simulink model "Fixed_Channel_Model_4_Channels"  (R2023a)
settings: Solver=ode23tb  StartTime=0.0  StopTime=3  RelTol=1e-3
libraries: dspfdesign x5, dspsrcs4 x4, dspvision x2
settings Model: Creator=zacha  LastModifiedBy=zacha
settings DebuggingCC: UnconnectedInputMsg=warning  UnconnectedOutputMsg=warning  UnconnectedLineMsg=warning
settings ModelReferenceCC: EnableRefExpFcnMdlSchedulingChecks=on
settings RTWCC: DLArmComputeVersion=19.05

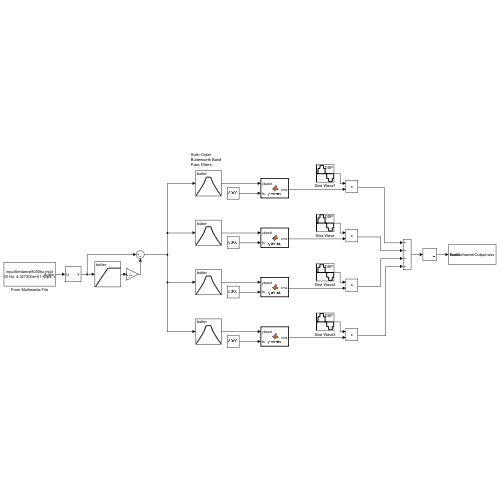
[thumbnail: Simulink's stored preview of the top-level diagram]
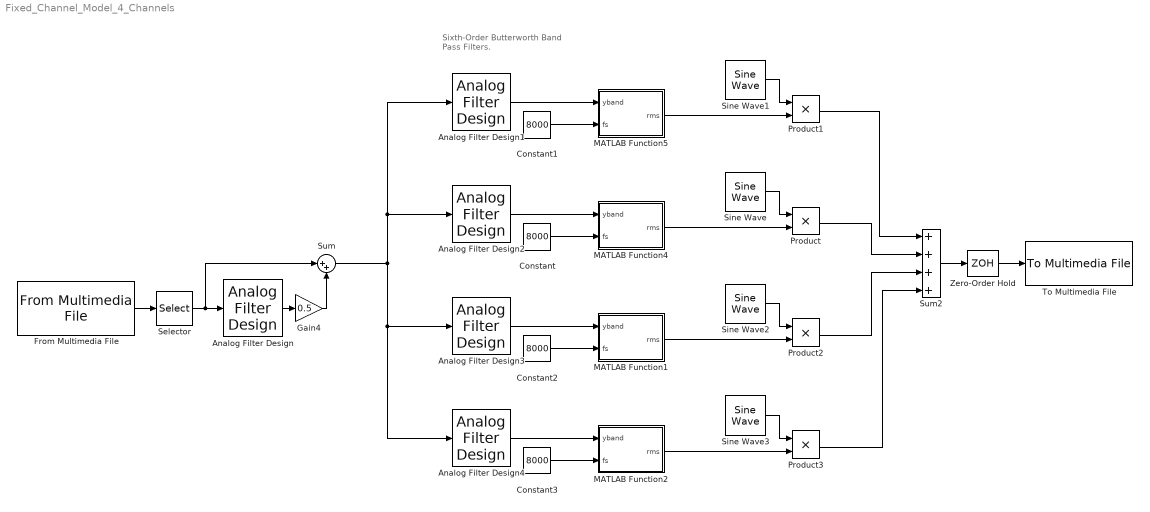
== system Fixed_Channel_Model_4_Channels ==
  note: Sixth-Order Butterworth Band Pass Filters.
  Analog Filter Design : dspfdesign/Analog Filter Design  method=Butterworth  filttype=Highpass  N=6  Wlo=7539.82236  Whi=80  Rp=2  Rs=40
  Analog Filter Design1 : dspfdesign/Analog Filter Design  method=Butterworth  filttype=Bandpass  N=6  Wlo=1570.796325  Whi=3476.7440370873  Rp=2  Rs=40
  Analog Filter Design2 : dspfdesign/Analog Filter Design  method=Butterworth  filttype=Bandpass  N=6  Wlo=3476.7440370873  Whi=7690.6188072  Rp=2  Rs=40
  Analog Filter Design3 : dspfdesign/Analog Filter Design  method=Butterworth  filttype=Bandpass  N=6  Wlo=7690.6188072  Whi=17032.45871124  Rp=2  Rs=40
  Analog Filter Design4 : dspfdesign/Analog Filter Design  method=Butterworth  filttype=Bandpass  N=6  Wlo=17032.45871124  Whi=37699.1118  Rp=2  Rs=40
  Constant{,1..3} (4 alike) : Constant  Value=8000
  From Multimedia File : dspvision/From Multimedia File  inputFilename=C:\Users\zacha\Desktop\Cochlear\Media\inputSentance8000hz.mp3  readRange=[1 Inf]  loop=on  numPlays=1  outputStreams=Audio only  videoDataType=single  audioDataType=double  inheritSampleTime=off  userDefinedSampleTime=1/8000  noAudioOutput=off  isIntensityVideo=off  fourcc=RGB  colorVideoFormat=Separate color signals  outputEOF=off  dataOrg=Column-major  audioFrameSize=1  computeAudioFrameSize=off  outSamplingMode=Sample based
      settings: LibrarySourceBlock=dspsrcs4/From Multimedia File
  Gain4 : Gain  Gain=0.5
  MATLAB Function1 : MATLAB Function  TreatAsAtomicUnit=on
  MATLAB Function2 : MATLAB Function  TreatAsAtomicUnit=on
  MATLAB Function4 : MATLAB Function  TreatAsAtomicUnit=on
  MATLAB Function5 : MATLAB Function  TreatAsAtomicUnit=on
  Product{,1..3} (4 alike) : Product
  Selector : Selector  NumberOfDimensions=2  InputPortWidth=3  IndexOptions=Select all,Index vector (dialog)  Indices=[2],1  OutputSizes=1,1
  Sine Wave : dspsrcs4/Sine Wave  Amplitude=1  Frequency=889.042915620874  Phase=0  SampleMode=Discrete  OutComplex=Real  CompMethod=Trigonometric fcn  TableSize=Speed  SampleTime=1/8000  SamplesPerFrame=1  ResetState=Restart at time zero  OutputFrames=off  dataType=double  wordLen=16  udDataType=sfix(16)  fracBitsMode=Best precision  numFracBits=15  OutDataTypeStr=double  LastOutDataTypeStr=double
  Sine Wave1 : dspsrcs4/Sine Wave  Amplitude=1  Frequency=401.670479925080  Phase=0  SampleMode=Discrete  OutComplex=Real  CompMethod=Trigonometric fcn  TableSize=Speed  SampleTime=1/8000  SamplesPerFrame=1  ResetState=Restart at time zero  OutputFrames=off  dataType=double  wordLen=16  udDataType=sfix(16)  fracBitsMode=Best precision  numFracBits=15  OutDataTypeStr=double  LastOutDataTypeStr=double
  Sine Wave2 : dspsrcs4/Sine Wave  Amplitude=1  Frequency=1967.77544111056  Phase=0  SampleMode=Discrete  OutComplex=Real  CompMethod=Trigonometric fcn  TableSize=Speed  SampleTime=1/8000  SamplesPerFrame=1  ResetState=Restart at time zero  OutputFrames=off  dataType=double  wordLen=16  udDataType=sfix(16)  fracBitsMode=Best precision  numFracBits=15  OutDataTypeStr=double  LastOutDataTypeStr=double
  Sine Wave3 : dspsrcs4/Sine Wave  Amplitude=1  Frequency=4355.40300541476  Phase=0  SampleMode=Discrete  OutComplex=Real  CompMethod=Trigonometric fcn  TableSize=Speed  SampleTime=1/8000  SamplesPerFrame=1  ResetState=Restart at time zero  OutputFrames=off  dataType=double  wordLen=16  udDataType=sfix(16)  fracBitsMode=Best precision  numFracBits=15  OutDataTypeStr=double  LastOutDataTypeStr=double
  Sum : Sum  Inputs=|++
  Sum2 : Sum  Inputs=++++
  To Multimedia File : dspvision/To Multimedia File  outputFilename=C:\Users\zacha\Desktop\Cochlear\Media\fixed4channelOutput.wav  streamSelection=Audio only  videoCompressor=None (uncompressed)  audioCompressor=None (uncompressed)  imagePorts=Separate color signals  fileType=WAV  audioDatatype=16-bit integer  fourcc=RGB  videoQuality=75  mj2000CompFactor=10
      settings: LibrarySourceBlock=dspsnks4/To Multimedia File
  Zero-Order Hold : ZeroOrderHold  SampleTime=-1
  wires:
  Analog Filter Design2/1 -> MATLAB Function4/1(yband)
  Constant/1 -> MATLAB Function4/2(fs)
  MATLAB Function4/1(rms) -> Product/2
  Sine Wave/1 -> Product/1
  Product/1 -> Sum2/2
  Product1/1 -> Sum2/1
  Sine Wave1/1 -> Product1/1
  Analog Filter Design1/1 -> MATLAB Function5/1(yband)
  MATLAB Function5/1(rms) -> Product1/2
  Constant1/1 -> MATLAB Function5/2(fs)
  Selector/1 -> Analog Filter Design/1, Sum/1
  Sine Wave2/1 -> Product2/1
  Analog Filter Design3/1 -> MATLAB Function1/1(yband)
  MATLAB Function1/1(rms) -> Product2/2
  Constant2/1 -> MATLAB Function1/2(fs)
  Sum/1 -> Analog Filter Design1/1, Analog Filter Design2/1, Analog Filter Design4/1, Analog Filter Design3/1
  Sine Wave3/1 -> Product3/1
  MATLAB Function2/1(rms) -> Product3/2
  Analog Filter Design4/1 -> MATLAB Function2/1(yband)
  Constant3/1 -> MATLAB Function2/2(fs)
  Product2/1 -> Sum2/3
  Product3/1 -> Sum2/4
  Sum2/1 -> Zero-Order Hold/1
  Zero-Order Hold/1 -> To Multimedia File/1
  From Multimedia File/1 -> Selector/1
  Analog Filter Design/1 -> Gain4/1
  Gain4/1 -> Sum/2

== matlab function Fixed_Channel_Model_4_Channels/MATLAB Function2 ==
  data: yband input; rms output; fs input
function rms = getrms(yband,fs)

    y = abs(yband); %rectifying it makes it sound bad

    [b,a] = butter(2,400/(fs/2));

    z = filter(b,a,y); %this filter also makes it sound bad

    windowsize = round(4/(1000/fs)); %rms computed every 4ms = windowsize samples

    [yupper,ylower] = envelope(yband,windowsize,'rms'); %changed to yband here

    %envelope(z,windowsize,'rms');

    rms = yupper;
end

== matlab function Fixed_Channel_Model_4_Channels/MATLAB Function4 ==
  data: yband input; rms output; fs input
function rms = getrms(yband,fs)

    y = abs(yband); %rectifying it makes it sound bad

    [b,a] = butter(2,400/(fs/2));

    z = filter(b,a,y); %this filter also makes it sound bad

    windowsize = round(4/(1000/fs)); %rms computed every 4ms = windowsize samples

    [yupper,ylower] = envelope(yband,windowsize,'rms'); %changed to yband here

    %envelope(z,windowsize,'rms');

    rms = yupper;
end

== matlab function Fixed_Channel_Model_4_Channels/MATLAB Function5 ==
  data: yband input; rms output; fs input
function rms = getrms(yband,fs)

    %y = abs(yband); %rectifying it makes it sound bad

    [b,a] = butter(2,400/(fs/2));

    %z = filter(b,a,y); %this filter also makes it sound bad

    windowsize = round(4/(1000/fs)); %rms computed every 4ms = windowsize samples

    [yupper,ylower] = envelope(yband,windowsize,'rms'); %changed to yband here

    %[yupper,ylower] = envelope(z,windowsize,'rms');

    rms = yupper;
end

== matlab function Fixed_Channel_Model_4_Channels/MATLAB Function1 ==
  data: yband input; rms output; fs input
function rms = getrms(yband,fs)

    y = abs(yband); %rectifying it makes it sound bad

    [b,a] = butter(2,400/(fs/2));

    z = filter(b,a,y); %this filter also makes it sound bad

    windowsize = round(4/(1000/fs)); %rms computed every 4ms = windowsize samples

    [yupper,ylower] = envelope(yband,windowsize,'rms'); %changed to yband here

    %envelope(z,windowsize,'rms');

    rms = yupper;
end
